simulink model "chap9_7sim"  (Simulink 7.7)
settings: Solver=ode45  StartTime=0.0  StopTime=30  FixedStep=0.001  RelTol=1e-3
settings Model: Creator=Administrator  LastModifiedBy=ljk  ExtModeTrigMode=oneshot  ExtModeArmWhenConnect=off
settings DataIOCC: LimitDataPoints=off  SignalLoggingName=sigsOut
settings OptimizationCC: BooleanDataType=off
settings DebuggingCC: SaveWithParameterizedLinksMsg=none  SignalResolutionControl=TryResolveAllWithWarning  SolverPrmCheckMsg=none  MultiTaskDSMMsg=warning  MultiTaskCondExecSysMsg=none  StrictBusMsg=None
settings HardwareCC: TargetUnknown=on
settings RTWCC: IncludeERTFirstTime=on

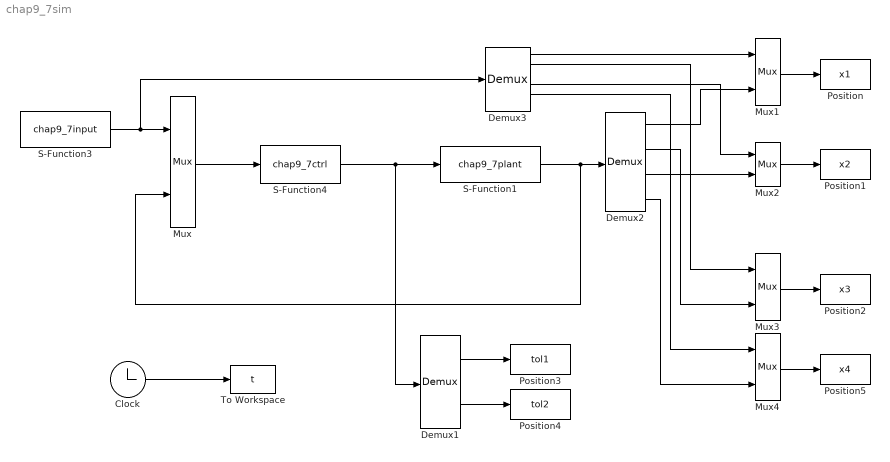
== system chap9_7sim ==
  Clock : Clock
      settings: Decimation=10
  Demux1 : Demux  Outputs=2
  Demux2 : Demux
  Demux3 : Demux  Outputs=6
  Mux{,1..4} (5 alike) : Mux  Inputs=2
  Position : ToWorkspace  VariableName=x1  SampleTime=-1  SaveFormat=Array
  Position1 : ToWorkspace  VariableName=x2  SampleTime=-1  SaveFormat=Array
  Position2 : ToWorkspace  VariableName=x3  SampleTime=-1  SaveFormat=Array
  Position3 : ToWorkspace  VariableName=tol1  SampleTime=-1  SaveFormat=Array
  Position4 : ToWorkspace  VariableName=tol2  SampleTime=-1  SaveFormat=Array
  Position5 : ToWorkspace  VariableName=x4  SampleTime=-1  SaveFormat=Array
  S-Function1 : S-Function  FunctionName=chap9_7plant  EnableBusSupport=off
  S-Function3 : S-Function  FunctionName=chap9_7input  EnableBusSupport=off
  S-Function4 : S-Function  FunctionName=chap9_7ctrl  EnableBusSupport=off
  To Workspace : ToWorkspace  VariableName=t  SampleTime=-1  SaveFormat=Array
  wires:
  Demux2/1 -> Mux1/2
  S-Function1/1 -> Mux/2, Demux2/1
  Demux1/1 -> Position3/1
  Demux1/2 -> Position4/1
  Demux3/1 -> Mux1/1
  Mux1/1 -> Position/1
  Mux2/1 -> Position1/1
  Demux3/4 -> Mux2/1
  Clock/1 -> To Workspace/1
  S-Function3/1 -> Mux/1, Demux3/1
  Mux/1 -> S-Function4/1
  S-Function4/1 -> S-Function1/1, Demux1/1
  Demux2/3 -> Mux2/2
  Demux3/2 -> Mux3/1
  Demux2/2 -> Mux3/2
  Demux3/5 -> Mux4/1
  Demux2/4 -> Mux4/2
  Mux3/1 -> Position2/1
  Mux4/1 -> Position5/1
